simulink model "main"  (R2023a)
settings: Solver=ode23s  StartTime=0.0  StopTime=inf  FixedStep=0.0001  RelTol=1e-3
undefined symbols (not defined in the file): J1, Jm, K, Km, l, La, Ra, smiData, X, Y, Z
libraries: sm_lib x14, nesl_utility x7, arduinolib x2, arduinosensorlib x2
settings Model: ExtModeTrigDuration=2  Creator=rocke  LastModifiedBy=Tarek
settings OptimizationCC: EnhancedBackFolding=on  PassReuseOutputArgsAs=Individual arguments  ZeroExternalMemoryAtStartup=off  ZeroInternalMemoryAtStartup=off  MaxStackSize=64  OptimizeBlockOrder=speed  DifferentSizesBufferReuse=on  OptimizationCustomize=off  EfficientTunableParamExpr=on
settings DebuggingCC: ParameterTunabilityLossMsg=error
settings HardwareCC: ProdBitPerPointer=32  ProdBitPerSizeT=32  ProdBitPerPtrDiffT=32  ProdLargestAtomicInteger=Long  ProdLargestAtomicFloat=Double  ProdWordSize=32  ProdHWDeviceType=ARM Compatible->ARM Cortex
settings SFSimCC: MATLABDynamicMemAlloc=off
settings RTWCC: Description=Embedded Coder  SystemTargetFile=ert.tlc  HardwareBoard=ESP32-WROOM(Arduino Compatible)  TLCOptions="-aInlineSetEventsForThisBaseRateFcn=TLC_FALSE -aSuppressMultiTaskScheduler=TLC_FALSE  -aRateBasedStepFcn=0"  TemplateMakefile=ert_default_tmf  Toolchain=ESP32  GPUComputeCapability=5.0
settings CodeAppCC: ForceParamTrailComments=on  IgnoreCustomStorageClasses=off  OperatorAnnotations=on  SimulinkDataObjDesc=on  SFDataObjDesc=on  InsertBlockDesc=on
settings ERTTargetCC: SupportContinuousTime=on  SupportVariableSizeSignals=on  ExtModeTransport=3  ExtModeStaticAlloc=on  ExtModeAutomaticAllocSize=off  ExtModeStaticAllocSize=65536  ExtModeMexFile=ext_xcp  ExtModeIntrfLevel=Level2 - Open

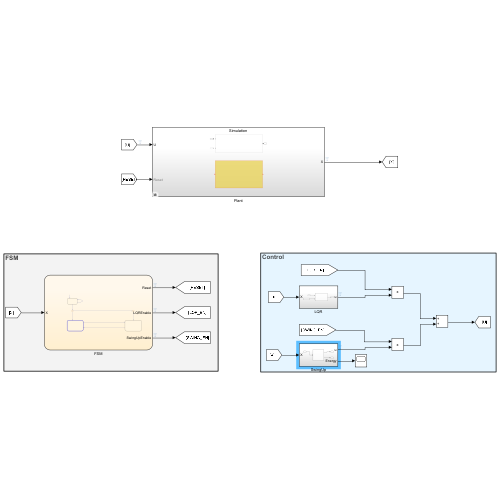
[thumbnail: Simulink's stored preview of the top-level diagram]
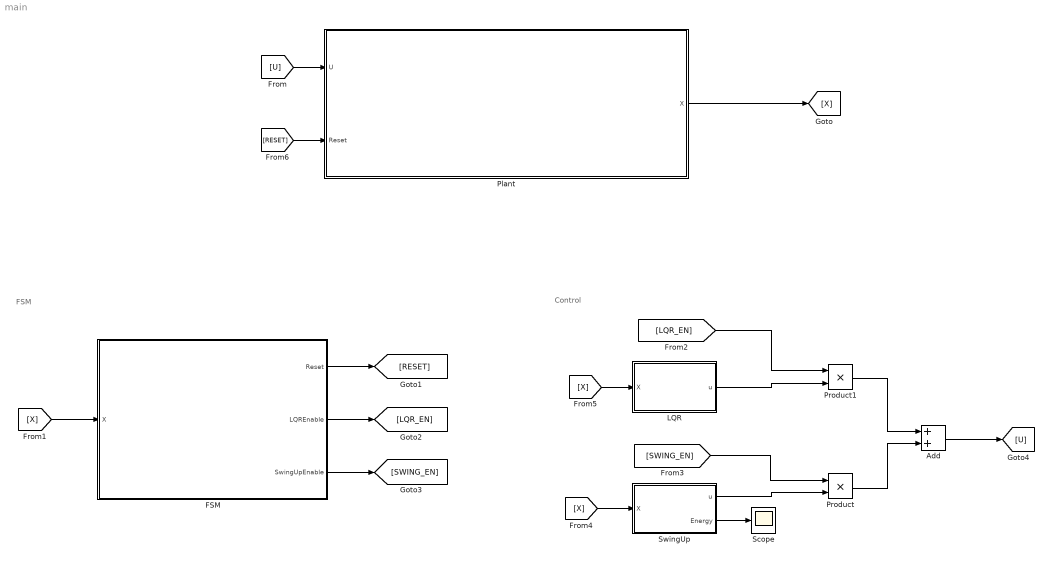
== system main ==
  note: Control
  note: FSM
  Add : Sum
  FSM : Stateflow chart  TreatAsAtomicUnit=on
  LQR : Subsystem
  Plant : Subsystem  Variant=on  VariantControlMode=label  VariantControl=Choice  LabelModeActiveChoice=Simulation
  Product : Product
  Product1 : Product
  Scope : Scope
  SwingUp : Subsystem
  wires:
  FSM/1(Reset) -> [RESET]
  FSM/2(LQREnable) -> [LQR_EN]
  FSM/3(SwingUpEnable) -> [SWING_EN]
  [X] -> SwingUp/1(X)
  [X] -> LQR/1(X)
  [U] -> Plant/1(U)
  [RESET] -> Plant/2(Reset)
  Plant/1(X) -> [X]
  [X] -> FSM/1(X)
  LQR/1(u) -> Product1/2
  [LQR_EN] -> Product1/1
  [SWING_EN] -> Product/1
  SwingUp/1(u) -> Product/2
  Add/1 -> [U]
  Product1/1 -> Add/1
  Product/1 -> Add/2
  SwingUp/2(Energy) -> Scope/1

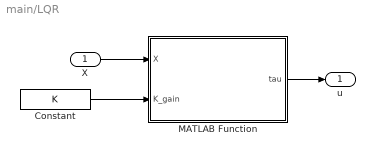
== system main/LQR ==
  X : Inport
  Constant : Constant  Value=K
  MATLAB Function : MATLAB Function  TreatAsAtomicUnit=on
  u : Outport
  wires:
  X/1 -> MATLAB Function/1(X)
  MATLAB Function/1(tau) -> u/1
  Constant/1 -> MATLAB Function/2(K_gain)

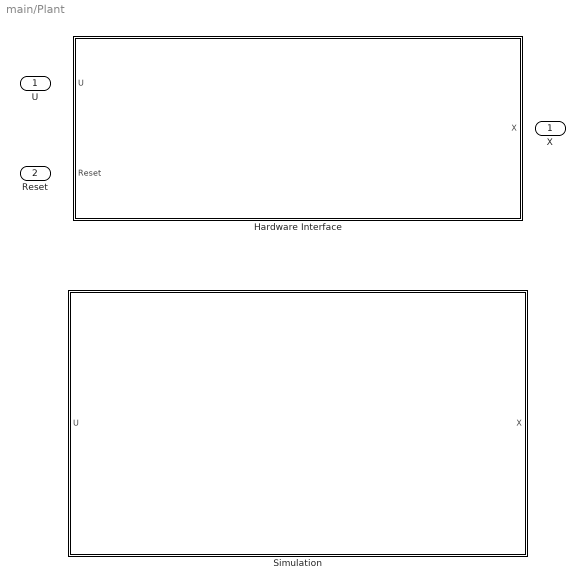
== system main/Plant ==
  U : Inport
  Reset : Inport  Port=2
  Hardware Interface : Subsystem  VariantControl=Hardware
  Simulation : Subsystem  VariantControl=Simulation
  X : Outport

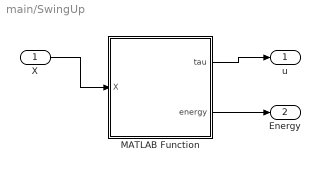
== system main/SwingUp ==
  X : Inport
  MATLAB Function : MATLAB Function  TreatAsAtomicUnit=on
  u : Outport
  Energy : Outport  Port=2
  wires:
  X/1 -> MATLAB Function/1(X)
  MATLAB Function/1(tau) -> u/1
  MATLAB Function/2(energy) -> Energy/1

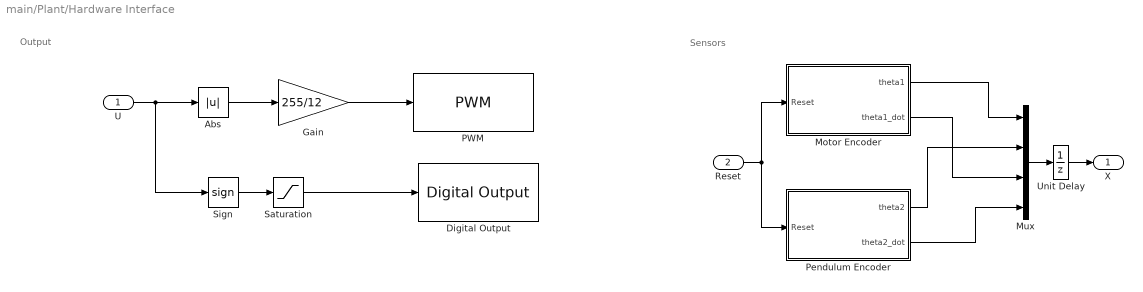
== system main/Plant/Hardware Interface ==
  note: Output
  note: Sensors
  U : Inport
  Reset : Inport  Port=2
  Abs : Abs  SaturateOnIntegerOverflow=off
  Digital Output : arduinolib/Digital Output  pinNumber=17  Direction=output  blockPlatform=arduino
  Gain : Gain  Gain=255/12
  Motor Encoder : Subsystem
  Mux : Mux
  PWM : arduinolib/PWM  pinNumber=5  frequencyType=Default  desiredFrequency=490.2  achievableFrequency=490.2
  Pendulum Encoder : Subsystem
  Saturation : Saturate  UpperLimit=1  LowerLimit=0  OutDataTypeStr=uint8
  Sign : Signum
  Unit Delay : UnitDelay  SampleTime=-1  HasFrameUpgradeWarning=on
  X : Outport
  wires:
  U/1 -> Sign/1, Abs/1
  Reset/1 -> Motor Encoder/1(Reset), Pendulum Encoder/1(Reset)
  Gain/1 -> PWM/1
  Pendulum Encoder/1(theta2) -> Mux/2
  Motor Encoder/1(theta1) -> Mux/1
  Saturation/1 -> Digital Output/1
  Motor Encoder/2(theta1_dot) -> Mux/3
  Pendulum Encoder/2(theta2_dot) -> Mux/4
  Abs/1 -> Gain/1
  Mux/1 -> Unit Delay/1
  Unit Delay/1 -> X/1
  Sign/1 -> Saturation/1

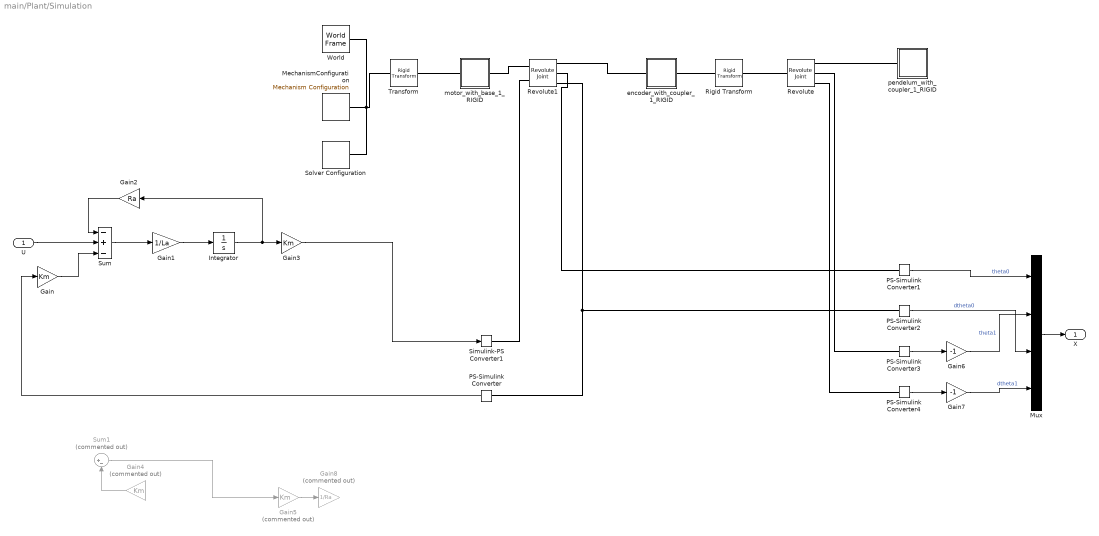
== system main/Plant/Simulation ==
  U : Inport
  Gain : Gain  Gain=Km
  Gain1 : Gain  Gain=1/La
  Gain2 : Gain  Gain=Ra
  Gain3 : Gain  Gain=Km
  Gain4 : Gain  Commented=on  Gain=Km
  Gain5 : Gain  Commented=on  Gain=Km
  Gain6 : Gain  Gain=-1
  Gain7 : Gain  Gain=-1
  Gain8 : Gain  Commented=on  Gain=1/Ra
  Integrator : Integrator
  MechanismConfiguration : sm_lib/Utilities/Mechanism Configuration  UniformGravity=Constant  GravityVector=[0 0 -9.80665]  GravityVectorUnits=m/s^2  LinearizationDelta=0.001  JointModeTransitionNonlinearIterations=2
  Mux : Mux
  PS-Simulink Converter{,1..4} (5 alike) : nesl_utility/PS-Simulink Converter  PhysicalDomain=network_engine_domain  SubClassName=ps_output  LeftPortType=input  RightPortType=output  PseudoPeriodic=off  Frequencies=[]  VectorFormat=inherit  Unit=inherit  AffineConversion=off
  Revolute : sm_lib/Joints/Revolute Joint  JointMode=Normal  SenseConstraintForce=off  SenseConstraintForceX=off  SenseConstraintForceY=off  SenseConstraintForceZ=off  SenseConstraintTorque=off  SenseConstraintTorqueX=off  SenseConstraintTorqueY=off  SenseConstraintTorqueZ=off  SenseTotalForce=off  SenseTotalForceX=off  SenseTotalForceY=off  SenseTotalForceZ=off  SenseTotalTorque=off  SenseTotalTorqueX=off  SenseTotalTorqueY=off  SenseTotalTorqueZ=off  CompositeWrenchDir=FollowerOnBase  CompositeWrenchFrame=BaseFrame  EquilibriumPosition=0  EquilibriumPositionUnits=deg  SpringStiffness=0  SpringStiffnessUnits=N*m/deg  DampingCoefficient=Beq_pend  DampingCoefficientUnits=N*m/(rad/s)  TorqueActuationMode=NoTorque  MotionActuationMode=ComputedMotion  SensePosition=on  SenseVelocity=on  SenseAcceleration=off  SenseTorqueForce=off  SenseLowerLimitTorqueForce=off  SenseUpperLimitTorqueForce=off  LowerLimitSpecify=off  LowerLimitBound=-360  LowerLimitBoundUnits=deg  LowerLimitStiffness=1e4  LowerLimitStiffnessUnits=N*m/deg  LowerLimitDamping=10  LowerLimitDampingUnits=N*m/(deg/s)  LowerLimitTransitionRegionWidth=0.1  LowerLimitTransitionRegionWidthUnits=deg  UpperLimitSpecify=off  UpperLimitBound=360  UpperLimitBoundUnits=deg  UpperLimitStiffness=1e4  UpperLimitStiffnessUnits=N*m/deg  UpperLimitDamping=10  UpperLimitDampingUnits=N*m/(deg/s)  UpperLimitTransitionRegionWidth=0.1  UpperLimitTransitionRegionWidthUnits=deg  PositionTargetSpecify=on  PositionTargetPriority=High  PositionTargetValue=0  PositionTargetValueUnits=deg  VelocityTargetSpecify=off  VelocityTargetPriority=High  VelocityTargetValue=0  VelocityTargetValueUnits=deg/s
  Revolute1 : sm_lib/Joints/Revolute Joint  JointMode=Normal  SenseConstraintForce=off  SenseConstraintForceX=off  SenseConstraintForceY=off  SenseConstraintForceZ=off  SenseConstraintTorque=off  SenseConstraintTorqueX=off  SenseConstraintTorqueY=off  SenseConstraintTorqueZ=off  SenseTotalForce=off  SenseTotalForceX=off  SenseTotalForceY=off  SenseTotalForceZ=off  SenseTotalTorque=off  SenseTotalTorqueX=off  SenseTotalTorqueY=off  SenseTotalTorqueZ=off  CompositeWrenchDir=FollowerOnBase  CompositeWrenchFrame=BaseFrame  EquilibriumPosition=0  EquilibriumPositionUnits=deg  SpringStiffness=0  SpringStiffnessUnits=N*m/deg  DampingCoefficient=Bm  DampingCoefficientUnits=N*m/(rad/s)  TorqueActuationMode=InputTorque  MotionActuationMode=ComputedMotion  SensePosition=on  SenseVelocity=on  SenseAcceleration=off  SenseTorqueForce=off  SenseLowerLimitTorqueForce=off  SenseUpperLimitTorqueForce=off  LowerLimitSpecify=off  LowerLimitBound=-90  LowerLimitBoundUnits=deg  LowerLimitStiffness=1e4  LowerLimitStiffnessUnits=N*m/deg  LowerLimitDamping=10  LowerLimitDampingUnits=N*m/(deg/s)  LowerLimitTransitionRegionWidth=0.1  LowerLimitTransitionRegionWidthUnits=deg  UpperLimitSpecify=off  UpperLimitBound=90  UpperLimitBoundUnits=deg  UpperLimitStiffness=1e4  UpperLimitStiffnessUnits=N*m/deg  UpperLimitDamping=10  UpperLimitDampingUnits=N*m/(deg/s)  UpperLimitTransitionRegionWidth=0.1  UpperLimitTransitionRegionWidthUnits=deg  PositionTargetSpecify=off  PositionTargetPriority=High  PositionTargetValue=0  PositionTargetValueUnits=deg  VelocityTargetSpecify=off  VelocityTargetPriority=High  VelocityTargetValue=0  VelocityTargetValueUnits=deg/s
  Rigid Transform : sm_lib/Frames and Transforms/Rigid Transform  TranslationMethod=None  TranslationStandardOffset=0  TranslationStandardOffsetUnits=m  TranslationStandardAxis=+Z  TranslationCartesianOffset=[0 0 0]  TranslationCartesianOffsetUnits=m  TranslationROffset=0  TranslationROffsetUnits=m  TranslationZOffset=0  TranslationZOffsetUnits=m  TranslationThetaOffset=0  TranslationThetaOffsetUnits=deg  RotationMethod=StandardAxis  RotationAngleUnits=deg  RotationStandardAxis=+Z  RotationAngle=-90  RotationArbitraryAxis=[0 0 1]  FollAlignAxisA=+X  BaseAlignAxisA=+Y  FollAlignAxisB=+Y  BaseAlignAxisB=+Z  RotationSequenceAxes=FollowerAxes  RotationSequence=XYX  RotationSequenceAngles=[0 0 0]  RotationSequenceAnglesUnits=deg  RotationMatrix=[1 0 0; 0 1 0; 0 0 1]  Quaternion=[1 0 0 0]
  Simulink-PS Converter1 : nesl_utility/Simulink-PS Converter  PhysicalDomain=network_engine_domain  SubClassName=ps_input  LeftPortType=input  RightPortType=output  PseudoPeriodic=off  Frequencies=[]  NoiseDistribution=none  NoiseParameters=[]  Unit=1  AffineConversion=off  FilteringAndDerivatives=provide  SimscapeFilterOrder=1  InputFilterTimeConstant=0.001  UdotUserProvided=0
  Solver Configuration : nesl_utility/Solver Configuration  PhysicalDomain=network_engine_domain  SubClassName=solver  LeftPortType=input  RightPortType=generic  Tones=[]  Harmonics=[]  SimulateNoise=off  Profile=off  UseLocalSampling=off  EnableSwitchedLinearOptims=on  FrequencyDomain=off  UseCCode=off  RelTol=0.001  AbsTol=0.001  MinStep=1e-09  ToWorkspace=off  RevertToSquareIcSolve=off  NumHomotopyIterations=100  PhasorMode=off  PhasorModeNumHarmonics=1  ConsistencySolver=NEWTON_XTOL_AFTER_FTOL  IndexReductionMethod=DerivativeReplacement  DoDC=off  ResidualTolerance=1e-09  ConsistencyTolSource=GLOBAL  ConsistencyAbsTol=0.001  ConsistencyRelTol=0.001  ConsistencyTolFactor=0.001  UseLocalSolver=off  LocalSolverChoice=NE_BACKWARD_EULER_ADVANCER  ResolveIndetEquations=on  FunctionEvalNumThread=1  LocalSolverSampleTime=0.001  DoFixedCost=off  MaxNonlinIter=3  MaxModeIter=2  ComputeImpulses=off  ImpulseIterations=2  LinearAlgebra=auto  LinearAlgebraNumThread=0  EquationFormulation=NE_TIME_EF  DelaysMemoryBudget=1024  AutomaticFiltering=on  FilteringTimeConstant=0.001  PartitionStorageMethod=AS_NEEDED  PartitionMemoryBudget=1024  PartitionMethod=ROBUST
  Sum : Sum  Inputs=-+-
  Sum1 : Sum  Commented=on  Inputs=|+-
  Transform : sm_lib/Frames and Transforms/Rigid Transform  TranslationMethod=Cartesian  TranslationStandardOffset=0  TranslationStandardOffsetUnits=m  TranslationStandardAxis=+Z  TranslationCartesianOffset=smiData.RigidTransform(6).translation  TranslationCartesianOffsetUnits=mm  TranslationROffset=0  TranslationROffsetUnits=m  TranslationZOffset=0  TranslationZOffsetUnits=m  TranslationThetaOffset=0  TranslationThetaOffsetUnits=deg  RotationMethod=ArbitraryAxis  RotationAngleUnits=rad  RotationStandardAxis=+Z  RotationAngle=smiData.RigidTransform(6).angle  RotationArbitraryAxis=smiData.RigidTransform(6).axis  FollAlignAxisA=+X  BaseAlignAxisA=+Y  FollAlignAxisB=+Y  BaseAlignAxisB=+Z  RotationSequenceAxes=FollowerAxes  RotationSequence=XYX  RotationSequenceAngles=[0 0 0]  RotationSequenceAnglesUnits=deg  RotationMatrix=[1 0 0; 0 1 0; 0 0 1]  Quaternion=[1 0 0 0]
  World : sm_lib/Frames and Transforms/World Frame
  encoder_with_coupler_1_RIGID : Subsystem
  motor_with_base_1_RIGID : Subsystem
  pendelum_with_coupler_1_RIGID : Subsystem
  X : Outport
  wires:
  Mux/1 -> X/1
  PS-Simulink Converter3/1 -> Gain6/1
  Gain7/1 -> Mux/4  "dtheta1"
  PS-Simulink Converter4/1 -> Gain7/1
  PS-Simulink Converter2/1 -> Mux/3  "dtheta0"
  PS-Simulink Converter1/1 -> Mux/1  "theta0"
  Gain6/1 -> Mux/2  "theta1"
  Gain/1 -> Sum/3
  Integrator/1 -> Gain3/1, Gain2/1
  Gain2/1 -> Sum/1
  Sum/1 -> Gain1/1
  Gain1/1 -> Integrator/1
  U/1 -> Sum/2
  Gain4/1 -> Sum1/2
  Gain5/1 -> Gain8/1
  Sum1/1 -> Gain5/1
  Gain3/1 -> Simulink-PS Converter1/1
  PS-Simulink Converter/1 -> Gain/1
  connections:
  PS-Simulink Converter/LConn1 -- PS-Simulink Converter2/LConn1 -- Revolute1/RConn3
  World/RConn1 -- Transform/LConn1 -- MechanismConfiguration/RConn1 -- Solver Configuration/RConn1
  Revolute1/RConn1 -- encoder_with_coupler_1_RIGID/LConn1
  Rigid Transform/RConn1 -- Revolute/LConn1
  Transform/RConn1 -- motor_with_base_1_RIGID/LConn1
  Simulink-PS Converter1/RConn1 -- Revolute1/LConn2
  PS-Simulink Converter4/LConn1 -- Revolute/RConn3
  PS-Simulink Converter3/LConn1 -- Revolute/RConn2
  PS-Simulink Converter1/LConn1 -- Revolute1/RConn2
  Revolute1/LConn1 -- motor_with_base_1_RIGID/RConn1
  Rigid Transform/LConn1 -- encoder_with_coupler_1_RIGID/RConn1
  Revolute/RConn1 -- pendelum_with_coupler_1_RIGID/LConn1

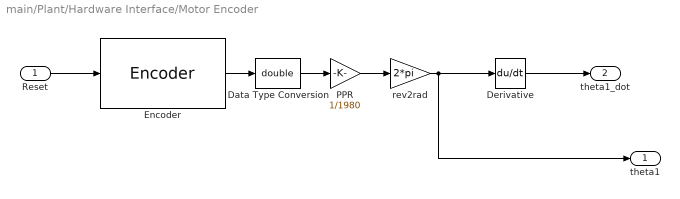
== system main/Plant/Hardware Interface/Motor Encoder ==
  Reset : Inport
  Data Type Conversion : DataTypeConversion  OutDataTypeStr=double  SaturateOnIntegerOverflow=off  RndMeth=Floor
  Derivative : Derivative
  Encoder : arduinosensorlib/Encoder  InputA=MOTOR_ENCODER_A  InputB=MOTOR_ENCODER_B  Mode=Reset by external signal  SampleTime=-1
  PPR : Gain  Gain=1/1980
  rev2rad : Gain  Gain=2*pi
  theta1 : Outport
  theta1_dot : Outport  Port=2
  wires:
  Data Type Conversion/1 -> PPR/1
  Derivative/1 -> theta1_dot/1
  PPR/1 -> rev2rad/1
  Encoder/1 -> Data Type Conversion/1
  Reset/1 -> Encoder/1
  rev2rad/1 -> theta1/1, Derivative/1

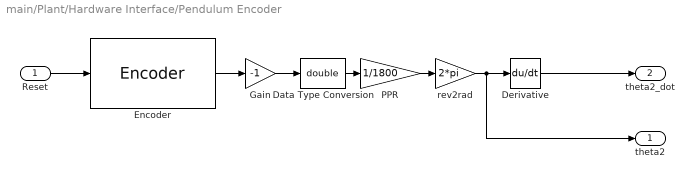
== system main/Plant/Hardware Interface/Pendulum Encoder ==
  Reset : Inport
  Data Type Conversion : DataTypeConversion  OutDataTypeStr=double  SaturateOnIntegerOverflow=off  RndMeth=Floor
  Derivative : Derivative
  Encoder : arduinosensorlib/Encoder  InputA=PENDULUM_ENCODER_A  InputB=PENDULUM_ENCODER_B  Mode=Reset by external signal  SampleTime=-1
  Gain : Gain  Gain=-1
  PPR : Gain  Gain=1/1800
  rev2rad : Gain  Gain=2*pi
  theta2 : Outport
  theta2_dot : Outport  Port=2
  wires:
  Data Type Conversion/1 -> PPR/1
  Derivative/1 -> theta2_dot/1
  PPR/1 -> rev2rad/1
  Encoder/1 -> Gain/1
  Reset/1 -> Encoder/1
  Gain/1 -> Data Type Conversion/1
  rev2rad/1 -> theta2/1, Derivative/1

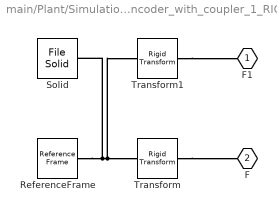
== system main/Plant/Simulation/encoder_with_coupler_1_RIGID ==
  ReferenceFrame : sm_lib/Frames and Transforms/Reference Frame
  Solid : sm_lib/Body Elements/File Solid  ExtGeomFileName=encoder_with_coupler_Default_sldprt.STEP  UnitType=FromFile  ExtGeomFileUnits=m  StepReaderType=HEX  ExportConvexHullGeometry=off  InertiaType=Custom  Mass=0.2  MassUnits=kg  CenterOfMass=[-182.67 0 243.85]  CenterOfMassUnits=mm  MomentsOfInertia=[0 Jm 0]  MomentsOfInertiaUnits=kg*m^2  ProductsOfInertia=[0 0 0]  ProductsOfInertiaUnits=kg*mm^2  BasedOnType=DensityFromFile  Density=1000  DensityUnits=kg/m^3  DoExposeReferenceFrame=on  SerializedFrames=<Frames/>  GraphicType=FromGeometry  MarkerShape=Sphere  MarkerSize=10  GraphicVisPropType=SimpleVisualProperties  GraphicDiffuseColor=smiData.Solid(1).color  GraphicSpecularColor=[0.5 0.5 0.5 1.0]  GraphicAmbientColor=[0.15 0.15 0.15 1.0]  GraphicEmissiveColor=[0.0 0.0 0.0 1.0]  GraphicShininess=75  GraphicOpacity=smiData.Solid(1).opacity
  Transform : sm_lib/Frames and Transforms/Rigid Transform  TranslationMethod=Cartesian  TranslationStandardOffset=0  TranslationStandardOffsetUnits=m  TranslationStandardAxis=+Z  TranslationCartesianOffset=smiData.RigidTransform(1).translation  TranslationCartesianOffsetUnits=mm  TranslationROffset=0  TranslationROffsetUnits=m  TranslationZOffset=0  TranslationZOffsetUnits=m  TranslationThetaOffset=0  TranslationThetaOffsetUnits=deg  RotationMethod=ArbitraryAxis  RotationAngleUnits=rad  RotationStandardAxis=+Z  RotationAngle=smiData.RigidTransform(1).angle  RotationArbitraryAxis=smiData.RigidTransform(1).axis  FollAlignAxisA=+X  BaseAlignAxisA=+Y  FollAlignAxisB=+Y  BaseAlignAxisB=+Z  RotationSequenceAxes=FollowerAxes  RotationSequence=XYX  RotationSequenceAngles=[0 0 0]  RotationSequenceAnglesUnits=deg  RotationMatrix=[1 0 0; 0 1 0; 0 0 1]  Quaternion=[1 0 0 0]
  Transform1 : sm_lib/Frames and Transforms/Rigid Transform  TranslationMethod=Cartesian  TranslationStandardOffset=0  TranslationStandardOffsetUnits=m  TranslationStandardAxis=+Z  TranslationCartesianOffset=smiData.RigidTransform(4).translation  TranslationCartesianOffsetUnits=mm  TranslationROffset=0  TranslationROffsetUnits=m  TranslationZOffset=0  TranslationZOffsetUnits=m  TranslationThetaOffset=0  TranslationThetaOffsetUnits=deg  RotationMethod=ArbitraryAxis  RotationAngleUnits=rad  RotationStandardAxis=+Z  RotationAngle=smiData.RigidTransform(4).angle  RotationArbitraryAxis=smiData.RigidTransform(4).axis  FollAlignAxisA=+X  BaseAlignAxisA=+Y  FollAlignAxisB=+Y  BaseAlignAxisB=+Z  RotationSequenceAxes=FollowerAxes  RotationSequence=XYX  RotationSequenceAngles=[0 0 0]  RotationSequenceAnglesUnits=deg  RotationMatrix=[1 0 0; 0 1 0; 0 0 1]  Quaternion=[1 0 0 0]
  F1 : PMIOPort  Side=Left
  F : PMIOPort  Port=2  Side=Right
  connections:
  Solid/RConn1 -- ReferenceFrame/RConn1 -- Transform/LConn1 -- Transform1/LConn1
  Transform/RConn1 -- F/RConn1
  Transform1/RConn1 -- F1/RConn1

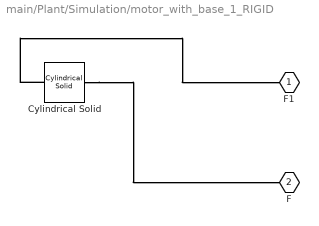
== system main/Plant/Simulation/motor_with_base_1_RIGID ==
  Cylindrical Solid : sm_lib/Body Elements/Cylindrical Solid  GraphicAmbientColor=[0.15 0.15 0.15 1.0]  BasedOnType=Density  CenterOfMass=[0 0 0]  CenterOfMassUnits=m  GraphicDiffuseColor=[0.5 0.5 0.5]  CylinderLength=0.1  CylinderLengthUnits=m  CylinderRadius=0.05  CylinderRadiusUnits=m  Density=1000  DensityUnits=kg/m^3  DoExposeReferenceFrame=off  GraphicEmissiveColor=[0.0 0.0 0.0 1.0]  ExportEntireGeometry=off  SerializedFrames=<Frames><Frame><Id>Frame1</Id><Value><Name>F1</Name><Origin><Source>GeometricFeature</Source><FeatureName>top surface</FeatureName></Origin><PrimaryAxis><DefinedDirection>+Z</DefinedDirection><Source>ReferenceFrame</Source><SourceDirection>+Z</SourceDirection><FeatureName></FeatureName></PrimaryAxis><SecondaryAxis><DefinedDirection>+X</DefinedDirection><Source>ReferenceFrame</Source><SourceDirection>+X</SourceDirection><FeatureName></FeatureName></SecondaryAxis></Value></Frame><Frame><Id>Frame2</Id><Value><Name>F2</Name><Origin><Source>GeometricFeature</Source><FeatureName>bottom surface</FeatureName></Origin><PrimaryAxis><DefinedDirection>+Z</DefinedDirection><Source>ReferenceFrame</Source><SourceDirection>+Z</SourceDirection><FeatureName></FeatureName></PrimaryAxis><SecondaryAxis><DefinedDirection>+X</DefinedDirection><Source>ReferenceFrame</Source><SourceDirection>+X</SourceDirection><FeatureName></FeatureName></SecondaryAxis></Value></Frame></Frames>  MarkerShape=Sphere  MarkerSize=10  GraphicType=FromGeometry  InertiaType=CalculateFromGeometry  Mass=1  MassUnits=kg  MomentsOfInertia=[1 1 1]  MomentsOfInertiaUnits=kg*m^2  GraphicOpacity=1.0  ProductsOfInertia=[0 0 0]  ProductsOfInertiaUnits=kg*m^2  GraphicShininess=75  GraphicSpecularColor=[0.5 0.5 0.5 1.0]  GraphicVisPropType=SimpleVisualProperties
  F1 : PMIOPort  Side=Left
  F : PMIOPort  Port=2  Side=Right
  connections:
  Cylindrical Solid/LConn1 -- F1/RConn1
  Cylindrical Solid/RConn1 -- F/RConn1

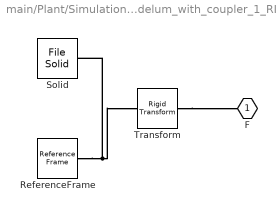
== system main/Plant/Simulation/pendelum_with_coupler_1_RIGID ==
  ReferenceFrame : sm_lib/Frames and Transforms/Reference Frame
  Solid : sm_lib/Body Elements/File Solid  ExtGeomFileName=pendelum_with_coupler_Default_sldprt.STEP  UnitType=FromFile  ExtGeomFileUnits=m  StepReaderType=HEX  ExportConvexHullGeometry=off  InertiaType=Custom  Mass=0.016  MassUnits=kg  CenterOfMass=[l 0 0.029]  CenterOfMassUnits=m  MomentsOfInertia=[0 0 J1]  MomentsOfInertiaUnits=kg*m^2  ProductsOfInertia=[0 0 0]  ProductsOfInertiaUnits=kg*mm^2  BasedOnType=DensityFromFile  Density=1000  DensityUnits=kg/m^3  DoExposeReferenceFrame=on  SerializedFrames=<Frames/>  GraphicType=FromGeometry  MarkerShape=Sphere  MarkerSize=10  GraphicVisPropType=SimpleVisualProperties  GraphicDiffuseColor=smiData.Solid(2).color  GraphicSpecularColor=[0.5 0.5 0.5 1.0]  GraphicAmbientColor=[0.15 0.15 0.15 1.0]  GraphicEmissiveColor=[0.0 0.0 0.0 1.0]  GraphicShininess=75  GraphicOpacity=smiData.Solid(2).opacity
  Transform : sm_lib/Frames and Transforms/Rigid Transform  TranslationMethod=Cartesian  TranslationStandardOffset=0  TranslationStandardOffsetUnits=m  TranslationStandardAxis=+Z  TranslationCartesianOffset=smiData.RigidTransform(2).translation  TranslationCartesianOffsetUnits=mm  TranslationROffset=0  TranslationROffsetUnits=m  TranslationZOffset=0  TranslationZOffsetUnits=m  TranslationThetaOffset=0  TranslationThetaOffsetUnits=deg  RotationMethod=ArbitraryAxis  RotationAngleUnits=rad  RotationStandardAxis=+Z  RotationAngle=smiData.RigidTransform(2).angle  RotationArbitraryAxis=smiData.RigidTransform(2).axis  FollAlignAxisA=+X  BaseAlignAxisA=+Y  FollAlignAxisB=+Y  BaseAlignAxisB=+Z  RotationSequenceAxes=FollowerAxes  RotationSequence=XYX  RotationSequenceAngles=[0 0 0]  RotationSequenceAnglesUnits=deg  RotationMatrix=[1 0 0; 0 1 0; 0 0 1]  Quaternion=[1 0 0 0]
  F : PMIOPort  Side=Left
  connections:
  Solid/RConn1 -- ReferenceFrame/RConn1 -- Transform/LConn1
  Transform/RConn1 -- F/RConn1

== matlab function main/LQR/MATLAB Function ==
  data: X input; tau output; K_gain input
function tau = lqr_balancer(X, K_gain)
    V_limit = 12;
    
    % Compute error relative to upright (pi)
    X_error = X;
    angle_err = (X(2) - pi);
    
    % Wrap error to [-pi, pi]
    angle_err = atan2(sin(angle_err), cos(angle_err));
    
    % If your sensor angle increases in the OPPOSITE direction of your model,
    % uncomment the next line:
    % angle_err = -angle_err;
    
    X_error(2) = angle_err;
    
    % LQR control law: u = -K * x_error
    u = -K_gain.' * X_error;  % K_gain must be 1x4 row vector
    
    tau = u;
    
    % Saturate
    tau = max(-V_limit, min(V_limit, tau));
end

== matlab function main/SwingUp/MATLAB Function ==
  settings: updateMethod=DISCRETE
  data: X input; tau output; energy output
function [tau, energy] = swing_up_controller(X)
% -------------------------------------------------------------------------
% 1. DEFINE PHYSICAL CONSTANTS
% -------------------------------------------------------------------------
    m1 = 0.016;           % Mass of pendulum (kg)
    l1 = 0.04;            % Distance to pendulum CoM (m)
    Jp_prime = 0.00006;   % Pendulum Inertia about pivot (kg*m^2)
    g = 9.81;             % Gravity (m/s^2)
    
    KE = 61;              % Energy Control Gain (MUST BE TUNED)
    BIAS = 2;           % Bias torque for kickstart when energy too low (TUNE THIS)
    E_BIAS_THRESHOLD = 0.0001; % Energy threshold below which bias is applied (TUNE THIS)
    
% -------------------------------------------------------------------------
% 2. EXTRACT STATE VARIABLES
% X = [theta0, theta1, theta0_dot, theta1_dot]
% theta1 = 0 → pendulum DOWN, theta1 = pi → pendulum UP
% -------------------------------------------------------------------------
    theta1 = X(2);           % Angle from DOWNWARD vertical
    theta1_dot = X(4);       % Angular velocity

% -------------------------------------------------------------------------
% 3. CALCULATE ENERGY USING STANDARD CONVENTION
% 
% STANDARD CONVENTION (with lowest point as reference):
%   Height above lowest point: h = l1*(1 - cos(theta1))  [theta1=0 is DOWN]
%   Potential Energy: V = m1*g*l1*(1 - cos(theta1))
%       → V = 0 at down (theta1 = 0)
%       → V = 2*m1*g*l1 at upright (theta1 = pi)
%   Kinetic Energy: T = 0.5*Jp_prime*theta1_dot^2
%   Total Energy: E = T + V
% -------------------------------------------------------------------------

% Target energy: pendulum upright (theta1 = pi) and stationary
    E_target = m1 * g * l1 * (1 - cos(pi));  % = 2*m1*g*l1
    
% Current energy
    V_current = m1 * g * l1 * (1 - cos(theta1));
    T_current = 0.5 * Jp_prime * theta1_dot^2;
    E_current = T_current + V_current;
    
% Energy error: positive when we need MORE energy
    E_error = E_target - E_current;

% -------------------------------------------------------------------------
% 4. ENERGY-BASED CONTROL LAW WITH BIAS KICKSTART
% 
% Standard swing-up control: tau = KE * E_error * theta1_dot * cos(theta1)
%   - Pumps energy when E_current < E_target
%   - The cos(theta1) term ensures we pump in phase with the motion
%   - At theta1 = pi/2, cos(theta1) = 0, so no pumping at horizontal
%   - Maximum pumping occurs near down position where |cos(theta1)| ≈ 1
%
% BIAS TERM: When energy is very low, add a constant bias to kickstart
%   - Only apply when E_current < E_BIAS_THRESHOLD
%   - Use sign(theta1_dot) to push in direction of motion
% -------------------------------------------------------------------------

    % Main energy pumping control
    tau = KE * E_error * theta1_dot * cos(theta1);
    
    % Add bias kickstart when energy is too low
    if E_current < E_BIAS_THRESHOLD
        tau = tau + BIAS * sign(theta1_dot);
        % If pendulum is stationary, give it a small push
        if abs(theta1_dot) < 0.01
            tau = tau + BIAS * sign(randn()); % Random direction push
        end
    end
    
    % Return energy error for monitoring
    energy = E_current;

% -------------------------------------------------------------------------
% 5. CLAMP TORQUE TO VOLTAGE LIMITS
% -------------------------------------------------------------------------
    V_limit = 12;
    tau = max(min(tau, V_limit), -V_limit);
end

== stateflow chart main/FSM ==
  note: If pendulum is moving while initializing, reset state.
  state INIT
  note: If 5 seconds elapsed without pendulum moving, reset angles and start control.
  state LQR
    entry:
    Reset=0;
    LQREnable=1;
    exit:
    LQREnable=0;
  state SwingUp
    entry:
    Reset=0;
    SwingUpEnable=1;
    exit:
    SwingUpEnable=0;
  (default) -> INIT
  INIT -> INIT [order 1] : [abs(X(4)) > 0.01]
  INIT -> (junction 5) [order 2] : [et > 5]{Reset=1;}
  (junction 5) -> (junction 10) [order 2] : [abs(wrapToPi(X(2) - pi)) >= pi/8 ]
  (junction 5) -> LQR [order 1] : [abs(wrapToPi(X(2) - pi)) < pi/13 ]
  (junction 10) -> SwingUp
  LQR -> SwingUp : [abs(wrapToPi(X(2) - pi)) >= pi/6 ]
  SwingUp -> LQR : [abs(wrapToPi(X(2) - pi)) < pi/13  ]
  data: X input; Reset output; LQREnable output; SwingUpEnable output
